simulink model "ex_kalman44"  (R2017a)
settings: Solver=FixedStepDiscrete  StartTime=0.0  StopTime=10  RelTol=1e-3  EnableMultiTasking=on
InitFcn:
  | load position.mat;
  | idx=[ 1 1 ;2 3 ;4 6 ;7 10 ;11 15 ;16 30 ;
  |      31 70 ;71 100 ;101 200 ;201 250 ;251 310];
  | LEN=length(idx);
  | t=(0:1:LEN-1)';
undefined symbols (not defined in the file or in its folder): FRAME_SIZE, position
CloseFcn:
  | rtwprivate ssgencode ModelCloseRequest ex_kalman33
settings Model: Creator=The MathWorks, Inc.  LastModifiedBy=The MathWorks, Inc.
settings DataIOCC: LimitDataPoints=on  SaveFormat=Structure
settings OptimizationCC: ExpressionDepthLimit=2147483647  LifeSpan=inf
settings DebuggingCC: UnderspecifiedInitializationDetection=Classic  MergeDetectMultiDrivingBlocksExec=none  SolverPrmCheckMsg=warning  FcnCallInpInsideContextMsg=warning  StateNameClashWarn=warning  SFUnexpectedBacktrackingDiag=warning  SFNoUnconditionalDefaultTransitionDiag=warning  SFExecutionAtInitializationDiag=none
settings HardwareCC: ProdBitPerPointer=32  ProdBitPerSizeT=32  ProdBitPerPtrDiffT=32  ProdLargestAtomicFloat=None  ProdIntDivRoundTo=Undefined  ProdEndianess=Unspecified  ProdWordSize=32  ProdHWDeviceType=32-bit Generic
settings ModelReferenceCC: PropagateSignalLabelsOutOfModel=off
settings SFSimCC: SimParseCustomCode=off
settings RTWCC: GenerateReport=on  LaunchReport=on
settings GRTTargetCC: TargetLangStandard=C89/C90 (ANSI)  GeneratePreprocessorConditionals=Disable all  CombineOutputUpdateFcns=off  GRTInterface=on
settings ConfigComp: CovMetricSettings=dw  CovHtmlReporting=on  CovSaveCumulativeToWorkspaceVar=on  CovSaveSingleToWorkspaceVar=on  CovExternalEMLEnable=off

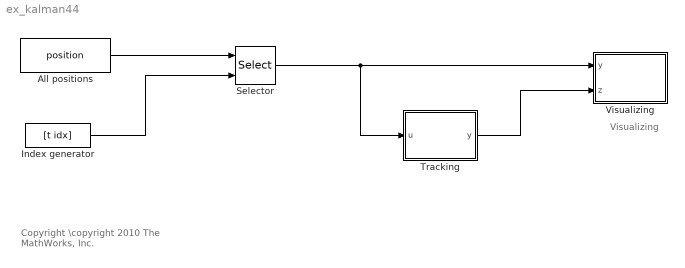
== system ex_kalman44 ==
  note: Visualizing
  note: Copyright \copyright 2010 The MathWorks, Inc.
  All positions : Constant  Value=position
  Index generator : FromWorkspace  VariableName=[t idx]  SampleTime=1  Interpolate=off  OutputAfterFinalValue=Holding final value
  Selector : Selector  NumberOfDimensions=2  InputPortWidth=2  IndexOptions=Select all,Starting and ending indices (port)  Indices=[1 3],2  OutputSizes=1,FRAME_SIZE
  Tracking : MATLAB Function  TreatAsAtomicUnit=on
  Visualizing : MATLAB Function  TreatAsAtomicUnit=on
  wires:
  All positions/1 -> Selector/1
  Index generator/1 -> Selector/2
  Selector/1 -> Visualizing/1(y), Tracking/1(u)
  Tracking/1(y) -> Visualizing/2(z)

== matlab function ex_kalman44/Visualizing ==
  data: y input; z input
function plot_me(y,z)
%#codegen
coder.extrinsic('figure','hold','plot_trajectory');
persistent h
if isempty(h)
  h=figure;
  hold;
end
plot_trajectory(y,z);
end

== matlab function ex_kalman44/Tracking ==
  data: u input; y output size=[2 100]
function y = kalman(u)
%#codegen

y = ex_kalman04(u);
